simulink model "Aero_Dynamics"  (Simulink 8.3)
settings: Solver=ode45  StartTime=0.0  StopTime=10.0  RelTol=1e-3
values from neighbouring files (symbols this model uses):
  AD = [0.05526	0.05526	0.05568	0.05804	0.06460	0.08210 ... (first row only)    [AirCraftData.m]
  Alpha0 = [0.143	0.143	0.122	-0.267	-0.627	0.120 ... (first row only)    [AirCraftData.m]
  CA = 3.451    [AirCraftData.m]    (also in AircraftTrim.m)
  CDmin = [0.03799	0.03799	0.03799	0.03799	0.03904	0.04277 ... (first row only)    [AirCraftData.m]
  CLAlpha = [0.1012	0.1021	0.1033	0.1051	0.1079	0.0976 ... (first row only)    [AirCraftData.m]
  Clbt0 = [-0.00147	-0.00148	-0.00149	-0.00153	-0.00158	-0.00171 ... (first row only)    [AirCraftData.m]
  Clbtaf = [0	0	0	0	0	0;0	 0	0	0	0	0]    [AirCraftData.m]
  ClDelA = [-0.003110	-0.003065	-0.003040	-0.003036	-0.003052	-0.003088 ... (first row only)    [AirCraftData.m]
  CLDelE = [0.00653	0.00668	0.00690	0.00724	0.00772	0.00846 ... (first row only)    [AirCraftData.m]
  ClDelR = [0.000584	0.000605	0.000638	0.000686	0.000760	0.000877 ... (first row only)    [AirCraftData.m]
  CLDM = [0.244	0.244	0.244	0.244	0.244	0.244 ... (first row only)    [AirCraftData.m]
  Clp0 = [-0.5510 	-0.5610 	-0.5767 	-0.6005 	-0.6224 	-0.6763 ... (first row only)    [AirCraftData.m]
  ClpAf = [0,0,0,0,0,0;0,0,0,0,0,0]    [AirCraftData.m]
  Clr0 = [0.1308 	0.1339 	0.1383 	0.1474 	0.1601 	0.1738 ... (first row only)    [AirCraftData.m]
  ClrAf = [0,0,0,0,0,0;0,0,0,0,0,0]    [AirCraftData.m]
  Cm0 = [0.2014	0.2017	0.2034	0.2083	0.2207	0.2475 ... (first row only)    [AirCraftData.m]
  CmAfdot = [-11.5890 	-12.0169 	-12.7558 	-13.8010 	-15.2088 	-16.2278 ... (first row only)    [AirCraftData.m]
  CmCl = [-0.3454	-0.3441	-0.3427	-0.3412	-0.3396	-0.3379 ... (first row only)    [AirCraftData.m]
  CmDelE = [-0.03554	-0.03651	-0.03802	-0.04028	-0.04365	-0.04798 ... (first row only)    [AirCraftData.m]
  Cmq0 = [-42.0260 	-42.2665 	-42.9499 	-44.8315 	-45.5877 	-46.0842 ... (first row only)    [AirCraftData.m]
  CN1A0 = [0.0740	0.0662	0.0605	0.0552	0.0554 ... (first row only)    [AirCraftData.m]
  Cnbt0 = [0.00180	0.00183	0.00187	0.00192	0.00200	0.00207 ... (first row only)    [AirCraftData.m]
  Cnbtaf = [-0.000030 	-0.000031 	-0.000031 	-0.000032 	-0.000033 	-0.000035 ... (first row only)    [AirCraftData.m]
  CnDelA0 = [-0.000180	-0.000178	-0.000176	-0.000176	-0.000177	-0.000179 ... (first row only)    [AirCraftData.m]
  CnDelAAf = [0	 0	0	0	0	0;0	 0	0	0	0	0]    [AirCraftData.m]
  CnDelR = [-0.002214	-0.002274	-0.002367	-0.002505	-0.002712	-0.003039 ... (first row only)    [AirCraftData.m]
  Cnp0 = [0.0521 	0.0532 	0.0571 	0.0601 	0.0636 	0.0664 ... (first row only)    [AirCraftData.m]
  CnpAf = [0,0,0,0,0,0;0,0,0,0,0,0]    [AirCraftData.m]
  Cnr = [-0.1810 	-0.1832 	-0.1855 	-0.1892 	-0.1933 	-0.1973 ... (first row only)    [AirCraftData.m]
  Cxh_Slip = [0.0000, 0.0045, 0.0089, 0.0132, 0.0174 ... (first row only)    [AirCraftData.m]
  Cybeta0 = [-0.01783	-0.01790	-0.01804	-0.01824	-0.01851	-0.01884 ... (first row only)    [AirCraftData.m]
  Cybtaf = [0 0 0 0 0 0;0 0 0 0 0 0]    [AirCraftData.m]
  CyDelA = [0.000287	0.000295	0.000307	0.000325	0.000351	0.000394 ... (first row only)    [AirCraftData.m]
  CyDelR = [0.004946	0.005035	0.005316	0.005791	0.006458	0.007318 ... (first row only)    [AirCraftData.m]
  Cyh_Slip = [0.0000, -0.0248, -0.0519, -0.0813, -0.1130 ... (first row only)    [AirCraftData.m]
  ETA_data = [0.729 0.727 0.72 0.71 0.877 0.858 0.855 0.853 0.857 0.862 0.87 0.796 ... (330 elements, 11x5x6)]    [ETA_data.mat]
  eul_0 = [0/57.3 0/57.3 0/57.3]    [AircraftTrim.m]
  flap = 0    [AircraftTrim.m]
  inertia = [  Ix      Iy     Iz  Ixz]    [AircraftTrim.m]
  mass = 54000    [Start.m]    (also in drl_simplified_dynamics.m)
  Vab_0 = [Vt 0 0]    [AircraftTrim.m]
  Wxyz_0 = [0 0 0]    [AircraftTrim.m]
  X = 1.06    [AircraftTrim.m]
  xme_0 = [0 0 -alt]    [AircraftTrim.m]
  Y = 1.177    [AircraftTrim.m]
undefined symbols (not defined in the file or in its folder): slselsubs, thrust_data
libraries: aerolibatmos2 x1, aerolibobsolete x1, aerolibutil x1
(part 2 of 2)

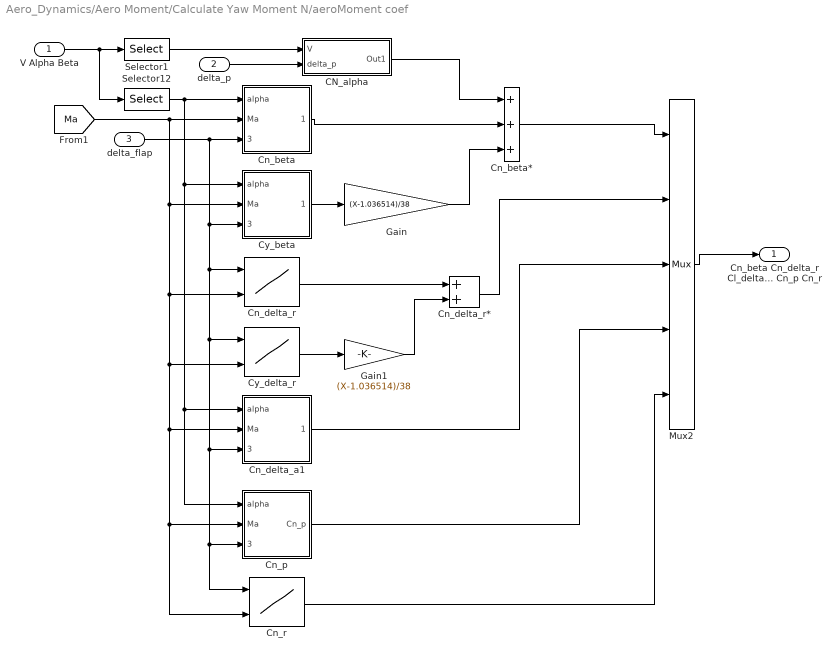
== system Aero_Dynamics/Aero Moment/Calculate Yaw Moment N/aeroMoment coef ==
  V Alpha Beta : Inport
  delta_p : Inport  Port=2
  delta_flap : Inport  Port=3
  CN_alpha : Subsystem
  Cn_beta : Subsystem
  Cn_beta* : Sum  Inputs=+++
  Cn_delta_a1 : Subsystem
  Cn_delta_r : Lookup2D  RowIndex=[0 6/57.3]  ColumnIndex=Mach_table  Table=CnDelR
  Cn_delta_r* : Sum
  Cn_p : Subsystem
  Cn_r : Lookup2D  RowIndex=[0 6/57.3]  ColumnIndex=Mach_table  Table=Cnr
  Cy_beta : Subsystem
  Cy_delta_r : Lookup2D  RowIndex=[0 6/57.3]  ColumnIndex=Mach_table  Table=CyDelR
  Gain : Gain  Gain=(X-1.036514)/38
  Gain1 : Gain  Gain=(X-1.036514)/38
  Mux2 : Mux  Inputs=5
  Selector1 : Selector  InputPortWidth=3  Indices=[1]  OutputSizes=[(-2)]
  Selector12 : Selector  InputPortWidth=3  Indices=[2]  OutputSizes=[(-2)]
  Cn_beta Cn_delta_r Cl_delta_a Cn_p Cn_r : Outport
  wires:
  [Ma] -> Cn_p/2(Ma), Cn_r/2, Cn_delta_a1/2(Ma), Cy_delta_r/2, Cn_delta_r/2, Cy_beta/2(Ma), Cn_beta/2(Ma)
  Mux2/1 -> Cn_beta Cn_delta_r Cl_delta_a Cn_p Cn_r/1
  delta_p/1 -> CN_alpha/2(delta_p)
  V Alpha Beta/1 -> Selector12/1, Selector1/1
  Cn_beta*/1 -> Mux2/1
  CN_alpha/1(Out1) -> Cn_beta*/1
  Cn_beta/1(Cnbeta) -> Cn_beta*/2
  Cy_beta/1(Cybeta) -> Gain/1
  Gain/1 -> Cn_beta*/3
  Cy_delta_r/1 -> Gain1/1
  Gain1/1 -> Cn_delta_r*/2
  Cn_delta_r/1 -> Cn_delta_r*/1
  Cn_delta_r*/1 -> Mux2/2
  Cn_delta_a1/1(Cn_delta_a) -> Mux2/3
  Cn_p/1(Cn_p) -> Mux2/4
  Cn_r/1 -> Mux2/5
  Selector12/1 -> Cn_beta/1(alpha), Cy_beta/1(alpha), Cn_delta_a1/1(alpha), Cn_p/1(alpha)
  Selector1/1 -> CN_alpha/1(V)
  delta_flap/1 -> Cn_beta/3(delta_flap), Cy_beta/3(delta_flap), Cn_delta_r/1, Cy_delta_r/1, Cn_delta_a1/3(delta_flap), Cn_p/3(delta_flap), Cn_r/1

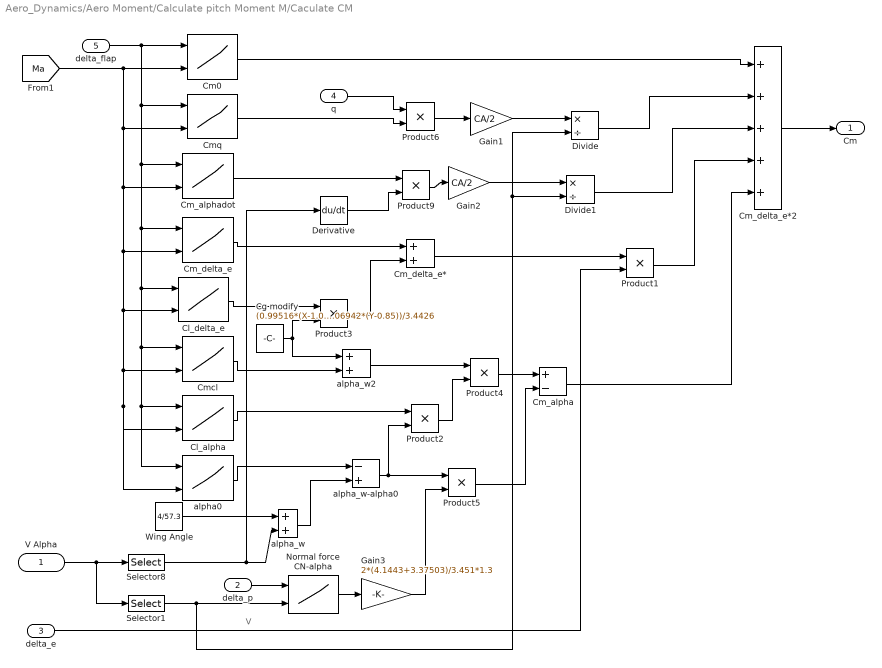
== system Aero_Dynamics/Aero Moment/Calculate pitch Moment M/Caculate CM  ==
  note: V
  " V Alpha" : Inport
  delta_p : Inport  Port=2
  delta_e : Inport  Port=3
  q : Inport  Port=4
  delta_flap : Inport  Port=5
  Cg modify : Constant  Value=(0.99516*(X-1.036514)-0.06942*(Y-0.85))/3.4426
  Cl_alpha : Lookup2D  RowIndex=[0 6/57.3]  ColumnIndex=Mach_table  Table=CLAlpha
  Cl_delta_e : Lookup2D  RowIndex=[0 6/57.3]  ColumnIndex=Mach_table  Table=CLDelE
  Cm0 : Lookup2D  RowIndex=[0 6/57.3]  ColumnIndex=Mach_table  Table=Cm0
  Cm_alpha : Sum  Inputs=+-
  Cm_alphadot : Lookup2D  RowIndex=[0 6/57.3]  ColumnIndex=Mach_table  Table=CmAfdot
  Cm_delta_e : Lookup2D  RowIndex=[0 6/57.3]  ColumnIndex=Mach_table  Table=CmDelE
  Cm_delta_e* : Sum
  Cm_delta_e*2 : Sum  Inputs=+++++
  Cmcl : Lookup2D  RowIndex=[0 6/57.3]  ColumnIndex=Mach_table  Table=CmCl
  Cmq : Lookup2D  RowIndex=[0 6/57.3]  ColumnIndex=Mach_table  Table=Cmq0
  Derivative : Derivative
  Divide : Product  Inputs=*/
  Divide1 : Product  Inputs=*/
  Gain1 : Gain  Gain=CA/2
  Gain2 : Gain  Gain=CA/2
  Gain3 : Gain  Gain=2*(4.1443+3.37503)/3.451*1.3
  Normal force CN-alpha : Lookup2D  RowIndex=[0.4,0.7,0.85,1,1.04]  ColumnIndex=[50,75,100,150,175]  Table=CN1A0
  Product{1..6,9} (7 alike) : Product  RndMeth=Zero
  Selector1 : Selector  InputPortWidth=2  Indices=[1]  OutputSizes=[(-2)]
  Selector8 : Selector  InputPortWidth=2  Indices=[2]  OutputSizes=[(-2)]
  Wing Angle : Constant  Value=4/57.3
  alpha0 : Lookup2D  RowIndex=[0 6/57.3]  ColumnIndex=Mach_table  Table=Alpha0
  alpha_w : Sum
  alpha_w-alpha0 : Sum  Inputs=-+
  alpha_w2 : Sum
  Cm : Outport
  wires:
  [Ma] -> Cl_alpha/2, alpha0/2, Cmcl/2, Cl_delta_e/2, Cm_delta_e/2, Cm_alphadot/2, Cmq/2, Cm0/2
  Cm_delta_e*2/1 -> Cm/1
  " V Alpha"/1 -> Selector8/1, Selector1/1
  Wing Angle/1 -> alpha_w/1
  Selector8/1 -> alpha_w/2, Derivative/1
  alpha0/1 -> alpha_w-alpha0/1
  alpha_w/1 -> alpha_w-alpha0/2
  alpha_w-alpha0/1 -> Product2/2, Product5/1
  Cl_alpha/1 -> Product2/1
  Normal force CN-alpha/1 -> Gain3/1
  Selector1/1 -> Divide/2, Divide1/2, Normal force CN-alpha/2
  alpha_w2/1 -> Product4/1
  Cg modify/1 -> Product3/2, alpha_w2/1
  Cl_delta_e/1 -> Product3/1
  Cm_delta_e/1 -> Cm_delta_e*/1
  Product3/1 -> Cm_delta_e*/2
  Product2/1 -> Product4/2
  Product4/1 -> Cm_alpha/1
  Gain3/1 -> Product5/2
  Product5/1 -> Cm_alpha/2
  Cmcl/1 -> alpha_w2/2
  delta_e/1 -> Product1/2
  Cm_delta_e*/1 -> Product1/1
  q/1 -> Product6/1
  Cmq/1 -> Product6/2
  Product6/1 -> Gain1/1
  Gain1/1 -> Divide/1
  Gain2/1 -> Divide1/1
  Product9/1 -> Gain2/1
  Derivative/1 -> Product9/2
  Cm_alphadot/1 -> Product9/1
  Cm0/1 -> Cm_delta_e*2/1
  Divide/1 -> Cm_delta_e*2/2
  Divide1/1 -> Cm_delta_e*2/3
  Product1/1 -> Cm_delta_e*2/4
  Cm_alpha/1 -> Cm_delta_e*2/5
  delta_p/1 -> Normal force CN-alpha/1
  delta_flap/1 -> Cm0/1, Cmq/1, Cm_alphadot/1, Cm_delta_e/1, Cl_delta_e/1, Cmcl/1, Cl_alpha/1, alpha0/1

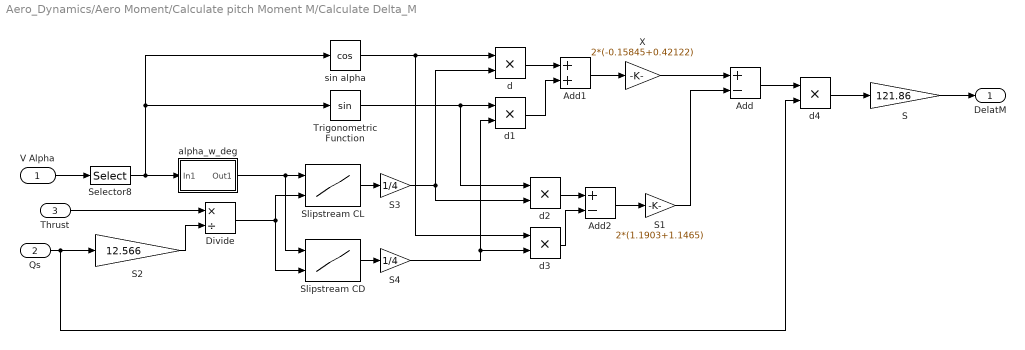
== system Aero_Dynamics/Aero Moment/Calculate pitch Moment M/Calculate Delta_M ==
  " V Alpha" : Inport
  Qs : Inport  Port=2
  Thrust : Inport  Port=3
  Add : Sum  Inputs=+-
  Add1 : Sum
  Add2 : Sum  Inputs=+-
  Divide : Product  Inputs=*/
  S : Gain  Gain=121.86
  S1 : Gain  Gain=2*(1.1903+1.1465)
  S2 : Gain  Gain=12.566
  S3 : Gain  Gain=1/4
  S4 : Gain  Gain=1/4
  Selector8 : Selector  InputPortWidth=2  Indices=[2]  OutputSizes=[(-2)]
  Slipstream CD : Lookup2D  RowIndex=[0,2,4,6,8,10,12,14,16,18]  ColumnIndex=[0,0.25,0.5,0.75,1]  Table=Cxh_Slip
  Slipstream CL : Lookup2D  RowIndex=[0,2,4,6,8,10,12,14,16 18]  ColumnIndex=[0 0.25 0.5 0.75 1]  Table=Cyh_Slip
  Trigonometric Function : Trigonometry
  X : Gain  Gain=2*(-0.15845+0.42122)
  alpha_w_deg : Subsystem
  d{,1..4} (5 alike) : Product  RndMeth=Zero
  sin alpha : Trigonometry  Operator=cos
  DelatM : Outport
  wires:
  Selector8/1 -> alpha_w_deg/1(In1), sin alpha/1, Trigonometric Function/1
  Qs/1 -> d4/2, S2/1
  Slipstream CL/1 -> S3/1
  sin alpha/1 -> d/1, d3/1
  d/1 -> Add1/1
  Add1/1 -> X/1
  Slipstream CD/1 -> S4/1
  Trigonometric Function/1 -> d1/1, d2/1
  d1/1 -> Add1/2
  X/1 -> Add/1
  S1/1 -> Add/2
  d2/1 -> Add2/1
  d3/1 -> Add2/2
  Add2/1 -> S1/1
  Add/1 -> d4/1
  d4/1 -> S/1
  S/1 -> DelatM/1
  " V Alpha"/1 -> Selector8/1
  S2/1 -> Divide/2
  Thrust/1 -> Divide/1
  Divide/1 -> Slipstream CL/2, Slipstream CD/2
  alpha_w_deg/1(Out1) -> Slipstream CL/1, Slipstream CD/1
  S3/1 -> d/2, d2/2
  S4/1 -> d1/2, d3/2

== system Aero_Dynamics/RusPlane/Calculate DCM & Euler Angles/phidot psidot thetadot ==
  note: p
      | q
      | r
  Wx Wy Wz : Inport
  phi theta psi : Inport  Port=2
  Mux1 : Mux  Inputs=[3 3 3]
  Mux2 : Mux  Inputs=3
  SinCos : aerolibobsolete/SinCos
  phidot : Fcn  Expr=u[1]+(u[2]*u[4]+u[3]*u[7])*(u[5]/u[8])
  psidot : Fcn  Expr=(u[2]*u[4]+u[3]*u[7])/u[8]
  thetadot : Fcn  Expr=u[2]*u[7]-u[3]*u[4]
  phidot thetadot psidot : Outport  InitialOutput=0
  wires:
  SinCos/2 -> Mux1/3
  SinCos/1 -> Mux1/2
  Mux2/1 -> phidot thetadot psidot/1
  phidot/1 -> Mux2/1
  thetadot/1 -> Mux2/2
  psidot/1 -> Mux2/3
  phi theta psi/1 -> SinCos/1
  Wx Wy Wz/1 -> Mux1/1
  Mux1/1 -> thetadot/1, phidot/1, psidot/1

== system Aero_Dynamics/Aero Moment/Calculate Roll Moment L/airdata/CN_alpha ==
  V : Inport
  delta_p : Inport  Port=2
  Gain3 : Gain  Gain=2*(0.5208+0.5909)/38
  Normal force CN-alpha : Lookup2D  RowIndex=[0.4,0.7,0.85,1,1.04]  ColumnIndex=[50,75,100,150,175]  Table=CN1A0
  Selector12 : Selector  InputPortWidth=3  Indices=[1]  OutputSizes=[(-2)]
  Out1 : Outport
  wires:
  Normal force CN-alpha/1 -> Gain3/1
  V/1 -> Selector12/1
  Gain3/1 -> Out1/1
  delta_p/1 -> Normal force CN-alpha/1
  Selector12/1 -> Normal force CN-alpha/2

== system Aero_Dynamics/Aero Moment/Calculate Roll Moment L/airdata/Cl_beta ==
  Ma : Inport
  alpha : Inport  Port=2
  delta_flap : Inport  Port=3
  Add1 : Sum
  Cl_beta0 : Lookup2D  RowIndex=[0 6/57.3]  ColumnIndex=Mach_table  Table=Clbt0
  Cl_beta_alpha : Lookup2D  RowIndex=[0 6/57.3]  ColumnIndex=Mach_table  Table=Clbtaf
  Product5 : Product  RndMeth=Zero
  C1beta : Outport
  wires:
  Cl_beta0/1 -> Add1/1
  Cl_beta_alpha/1 -> Product5/1
  Product5/1 -> Add1/2
  Ma/1 -> Cl_beta0/2, Cl_beta_alpha/2
  Add1/1 -> C1beta/1
  alpha/1 -> Product5/2
  delta_flap/1 -> Cl_beta0/1, Cl_beta_alpha/1

== system Aero_Dynamics/Aero Moment/Calculate Roll Moment L/airdata/Cl_p ==
  alpha : Inport
  Ma : Inport  Port=2
  delta_flap : Inport  Port=3
  Add1 : Sum
  Cl_p0 : Lookup2D  RowIndex=[0 6/57.3]  ColumnIndex=Mach_table  Table=Clp0
  Clp_alpha : Lookup2D  RowIndex=[0 6/57.3]  ColumnIndex=Mach_table  Table=ClpAf
  Product5 : Product  RndMeth=Zero
  Cl_p : Outport
  wires:
  alpha/1 -> Product5/2
  Add1/1 -> Cl_p/1
  Ma/1 -> Cl_p0/2, Clp_alpha/2
  Product5/1 -> Add1/2
  Clp_alpha/1 -> Product5/1
  Cl_p0/1 -> Add1/1
  delta_flap/1 -> Cl_p0/1, Clp_alpha/1

== system Aero_Dynamics/Aero Moment/Calculate Roll Moment L/airdata/Cl_r ==
  alpha : Inport
  Ma : Inport  Port=2
  delta_flap : Inport  Port=3
  Add1 : Sum
  Cl_r0 : Lookup2D  RowIndex=[0 6/57.3]  ColumnIndex=Mach_table  Table=Clr0
  Clr_alpha : Lookup2D  RowIndex=[0 6/57.3]  ColumnIndex=Mach_table  Table=ClrAf
  Product5 : Product  RndMeth=Zero
  Cl_r : Outport
  wires:
  Cl_r0/1 -> Add1/1
  Clr_alpha/1 -> Product5/1
  Product5/1 -> Add1/2
  Ma/1 -> Cl_r0/2, Clr_alpha/2
  Add1/1 -> Cl_r/1
  alpha/1 -> Product5/2
  delta_flap/1 -> Cl_r0/1, Clr_alpha/1

== system Aero_Dynamics/Aero Moment/Calculate Roll Moment L/airdata/Cy_beta ==
  alpha : Inport
  delta_flap : Inport  Port=2
  Ma : Inport  Port=3
  Add1 : Sum
  Cy_beta0 : Lookup2D  RowIndex=[0 6/57.3]  ColumnIndex=Mach_table  Table=Cybeta0
  Cy_beta_alpha : Lookup2D  RowIndex=[0 6/57.3]  ColumnIndex=Mach_table  Table=Cybtaf
  Product5 : Product  RndMeth=Zero
  Cybeta : Outport
  wires:
  Cy_beta0/1 -> Add1/1
  Cy_beta_alpha/1 -> Product5/1
  Product5/1 -> Add1/2
  Ma/1 -> Cy_beta0/2, Cy_beta_alpha/2
  Add1/1 -> Cybeta/1
  alpha/1 -> Product5/2
  delta_flap/1 -> Cy_beta0/1, Cy_beta_alpha/1

== system Aero_Dynamics/Aero Moment/Calculate Yaw Moment N/aeroMoment coef/CN_alpha ==
  V : Inport
  delta_p : Inport  Port=2
  Gain3 : Gain  Gain=-2*(4.1443+3.37503)/38
  Normal force CN-alpha : Lookup2D  RowIndex=[0.4,0.7,0.85,1,1.04]  ColumnIndex=[50,75,100,150,175]  Table=CN1A0
  Out1 : Outport
  wires:
  Normal force CN-alpha/1 -> Gain3/1
  Gain3/1 -> Out1/1
  delta_p/1 -> Normal force CN-alpha/1
  V/1 -> Normal force CN-alpha/2

== system Aero_Dynamics/Aero Moment/Calculate Yaw Moment N/aeroMoment coef/Cn_beta ==
  alpha : Inport
  Ma : Inport  Port=2
  delta_flap : Inport  Port=3
  Add1 : Sum
  Add2 : Sum  Inputs=+-
  Cn_beta0 : Lookup2D  RowIndex=[0 6/57.3]  ColumnIndex=Mach_table  Table=Cnbt0
  Cn_beta_alpha : Lookup2D  RowIndex=[0 6/57.3]  ColumnIndex=Mach_table  Table=Cnbtaf
  Constant : Constant  Value=4/57.3
  Product5 : Product  RndMeth=Zero
  Cnbeta : Outport
  wires:
  Add1/1 -> Cnbeta/1
  Ma/1 -> Cn_beta0/2, Cn_beta_alpha/2
  Product5/1 -> Add1/2
  Cn_beta_alpha/1 -> Product5/1
  Cn_beta0/1 -> Add1/1
  delta_flap/1 -> Cn_beta0/1, Cn_beta_alpha/1
  alpha/1 -> Add2/1
  Add2/1 -> Product5/2
  Constant/1 -> Add2/2

== system Aero_Dynamics/Aero Moment/Calculate Yaw Moment N/aeroMoment coef/Cn_delta_a1 ==
  alpha : Inport
  Ma : Inport  Port=2
  delta_flap : Inport  Port=3
  Add1 : Sum
  Cn_delta_a0 : Lookup2D  RowIndex=[0 6/57.3]  ColumnIndex=Mach_table  Table=CnDelA0
  Cn_delta_alpha : Lookup2D  RowIndex=[0 6/57.3]  ColumnIndex=Mach_table  Table=CnDelAAf
  Product5 : Product  RndMeth=Zero
  Cn_delta_a : Outport
  wires:
  Cn_delta_a0/1 -> Add1/1
  Cn_delta_alpha/1 -> Product5/1
  Product5/1 -> Add1/2
  Ma/1 -> Cn_delta_a0/2, Cn_delta_alpha/2
  Add1/1 -> Cn_delta_a/1
  alpha/1 -> Product5/2
  delta_flap/1 -> Cn_delta_a0/1, Cn_delta_alpha/1

== system Aero_Dynamics/Aero Moment/Calculate Yaw Moment N/aeroMoment coef/Cn_p ==
  alpha : Inport
  Ma : Inport  Port=2
  delta_flap : Inport  Port=3
  Add1 : Sum
  Cn_p0 : Lookup2D  RowIndex=[0 6/57.3]  ColumnIndex=Mach_table  Table=Cnp0
  Cnp_alpha : Lookup2D  RowIndex=[0 6/57.3]  ColumnIndex=Mach_table  Table=CnpAf
  Product5 : Product  RndMeth=Zero
  Cn_p : Outport
  wires:
  alpha/1 -> Product5/2
  Add1/1 -> Cn_p/1
  Ma/1 -> Cn_p0/2, Cnp_alpha/2
  Product5/1 -> Add1/2
  Cnp_alpha/1 -> Product5/1
  Cn_p0/1 -> Add1/1
  delta_flap/1 -> Cn_p0/1, Cnp_alpha/1

== system Aero_Dynamics/Aero Moment/Calculate Yaw Moment N/aeroMoment coef/Cy_beta ==
  alpha : Inport
  Ma : Inport  Port=2
  delta_flap : Inport  Port=3
  Add1 : Sum
  Cy_beta0 : Lookup2D  RowIndex=[0 6/57.3]  ColumnIndex=Mach_table  Table=Cybeta0
  Cy_beta_alpha : Lookup2D  RowIndex=[0 6/57.3]  ColumnIndex=Mach_table  Table=Cybtaf
  Product5 : Product  RndMeth=Zero
  Cybeta : Outport
  wires:
  Cy_beta0/1 -> Add1/1
  Cy_beta_alpha/1 -> Product5/1
  Product5/1 -> Add1/2
  Ma/1 -> Cy_beta_alpha/2, Cy_beta0/2
  Add1/1 -> Cybeta/1
  alpha/1 -> Product5/2
  delta_flap/1 -> Cy_beta0/1, Cy_beta_alpha/1

== system Aero_Dynamics/Aero Moment/Calculate pitch Moment M/Calculate Delta_M/alpha_w_deg ==
  In1 : Inport
  Constant : Constant  Value=4
  S3 : Gain  Gain=57.3
  Subtract : Sum
  Out1 : Outport
  wires:
  S3/1 -> Subtract/1
  Constant/1 -> Subtract/2
  In1/1 -> S3/1
  Subtract/1 -> Out1/1
